simulink subsystem "PropulsionSystemDriveline"  (R2024b)
settings: Solver=VariableStepAuto  StartTime=0.0  StopTime=10.0  RelTol=1e-3
model mask{RotorArm=0, Kp=0, Ki=0, Kd=0, N=0}
  mask prompts: RotorArm "Rotor Arm"
settings Model: Creator=jjha  LastModifiedBy=jjha
settings RTWCC: GPUComputeCapability=3.5

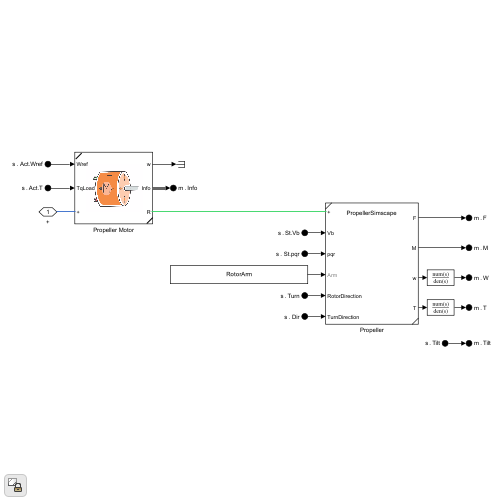
[thumbnail: Simulink's stored preview of the top-level diagram]
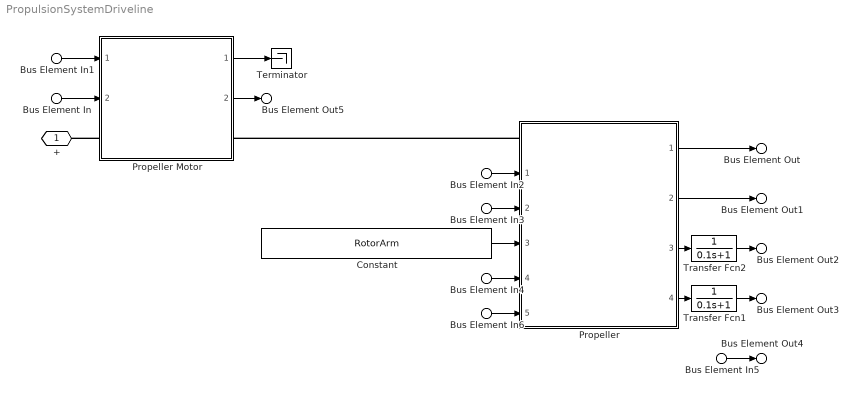
== system PropulsionSystemDriveline ==
  Bus Element In4 : Inport  PortName=s  Element=Turn
  Bus Element In5 : Inport  PortName=s  Element=Tilt
  Bus Element In3 : Inport  PortName=s  Element=St.pqr
  Bus Element In2 : Inport  PortName=s  Element=St.Vb
  Bus Element In1 : Inport  PortName=s  Element=Act.Wref
  Bus Element In : Inport  PortName=s  Element=Act.T
  Bus Element In6 : Inport  PortName=s  Element=Dir
  Constant : Constant  Value=RotorArm
  Propeller : Subsystem  ReferencedSubsystem=PropellerSimscape
      settings: PortSchema="{\"entries\":[{\"content\":{\"sides\":[{\"content\":{\"connectorIds\":[\"LConn1\",\"In1\",\"In2\",\"In3\",\"In4\",\"In5\"]},\"type\":\"ConnectorPlacement.EquallySpacedRectSide\",\"uuid\":\"389d9263-9c95-4b6f-a6f9-dc4a7ce75646\"},{\"content\":{\"connectorIds\":[\"Out1\",\"Out2\",\"Out3\",\"Out4\"],\"side\":\"RIGHT\"},\"type\":\"ConnectorPlacement.EquallySpacedRectSide\",\"uuid\":\"43fbe599-c819-4cc7-a4ff-3295ea5fa308\"},{\"content\":{\"side\":\"TOP\"},\"type\":\"ConnectorPlacement.EquallySpacedRectSide\",\"uuid\":\"cb4b893a-d6f1-4e6b-9f7f-7fcdd3ed6ff2\"}]},\"type\":\"ConnectorPlacement.EquallySpacedConnector\",\"uuid\":\"e6528a26-12d1-410f-874c-0dd6e5265179\"}],\"packageUris\":[\"http://schema.mathworks.com/mf0/Connector/R2020b\"],\"version\":\"1.0\"}"
  Propeller Motor : Subsystem  ReferencedSubsystem=PropulsionMotor  Kp=Kp  Ki=Ki  Kd=Kd  N=N
  Terminator : Terminator
  Transfer Fcn1 : TransferFcn  Denominator=[0.1 1]  AbsoluteTolerance=1e-3
  Transfer Fcn2 : TransferFcn  Denominator=[0.1 1]  AbsoluteTolerance=1e-3
  + : PMIOPort  Side=Right
  Bus Element Out : Outport  PortName=m  Element=F
  Bus Element Out1 : Outport  PortName=m  Element=M
  Bus Element Out2 : Outport  PortName=m  Element=W
  Bus Element Out3 : Outport  PortName=m  Element=T
  Bus Element Out4 : Outport  PortName=m  Element=Tilt
  Bus Element Out5 : Outport  PortName=m  Element=Info
  wires:
  Bus Element In4/1 -> Propeller/4
  Constant/1 -> Propeller/3
  Bus Element In6/1 -> Propeller/5
  Bus Element In3/1 -> Propeller/2
  Bus Element In1/1 -> Propeller Motor/1
  Propeller/1 -> Bus Element Out/1
  Propeller/2 -> Bus Element Out1/1
  Propeller/3 -> Transfer Fcn2/1
  Propeller/4 -> Transfer Fcn1/1
  Transfer Fcn2/1 -> Bus Element Out2/1
  Bus Element In5/1 -> Bus Element Out4/1
  Bus Element In2/1 -> Propeller/1
  Bus Element In/1 -> Propeller Motor/2
  Propeller Motor/1 -> Terminator/1
  Propeller Motor/2 -> Bus Element Out5/1
  Transfer Fcn1/1 -> Bus Element Out3/1
  connections:
  Propeller Motor/LConn1 -- +/RConn1
  Propeller/LConn1 -- Propeller Motor/RConn1
